simulink model "FOC IM"  (R2016a)
settings: Solver=VariableStepAuto  StartTime=0.0  StopTime=inf  FixedStep=0.000000001  RelTol=1e-4  SampleTimeConstraint=Specified
InitFcn:
  | P=2;
  | f=50;
  | we=2*pi*f;
  | rs=1.77;
  | lls=0.0139;
  | rr=1.34;
  | llr=0.0121;
  | tow=llr/rr;
  | lm=0.3687;
  | lad=1/(1/lm+1/lls+1/llr);
  | laq=lad;
  | Tl=0.1;
  | B=0.0000;
  | J=0.001;
  | Vdc=1000;
libraries: simulink x3
settings Model: Creator=moham  LastModifiedBy=moham
settings SolverCC: AutoInsertRateTranBlk=on
settings DataIOCC: ReturnWorkspaceOutputs=on
settings DebuggingCC: ArtificialAlgebraicLoopMsg=none  SFUnexpectedBacktrackingDiag=error  SFNoUnconditionalDefaultTransitionDiag=error
settings SFSimCC: SimUseLocalCustomCode=on
settings RTWCC: RTWUseLocalCustomCode=on
settings GRTTargetCC: TargetLangStandard=C99 (ISO)
settings ConfigComp: CovMetricSettings=dwe  CovSaveCumulativeToWorkspaceVar=off  CovSaveSingleToWorkspaceVar=off  CovExternalEMLEnable=on

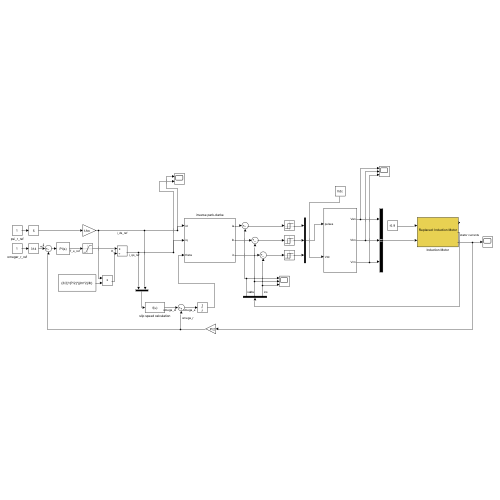
[thumbnail: Simulink's stored preview of the top-level diagram]
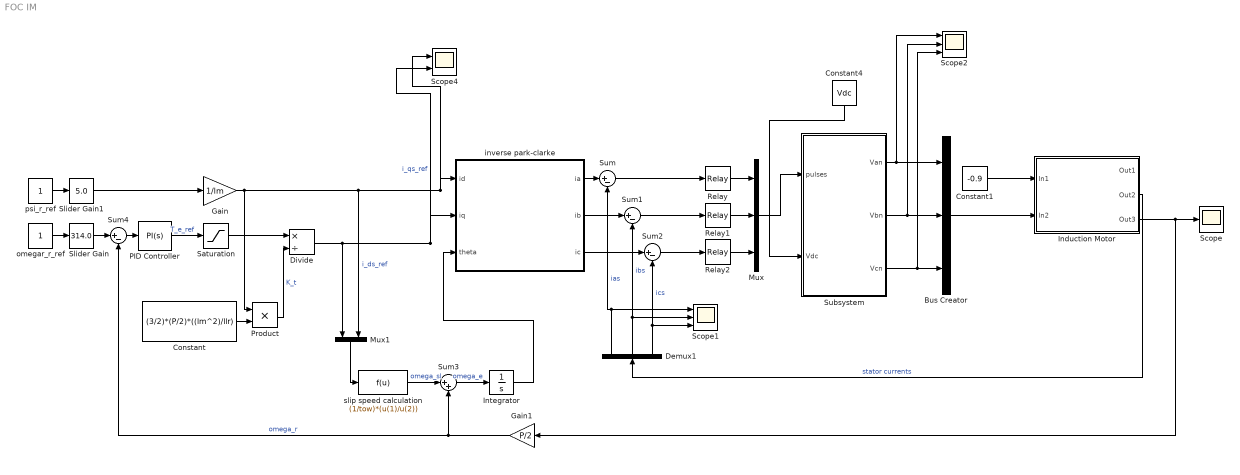
== system FOC IM ==
  Bus Creator : BusCreator  Inputs=3
  Constant : Constant  Value=(3/2)*(P/2)*((lm^2)/llr)
  Constant1 : Constant  Value=-0.9
  Constant4 : Constant  Value=Vdc
  Demux1 : Demux  Outputs=3
  Divide : Product  Inputs=*/
  Gain : Gain  Gain=1/lm
  Gain1 : Gain  Gain=P/2
  Induction Motor : Subsystem  Description=Replaced Block  mask(Replaced Block){}
      mask help: This block has been replaced with an empty subsystem because it used functionality that is unavailable in Simulink R2016a.
      mask Display: fprintf('Replaced: %s\n','Induction Motor')
  Integrator : Integrator
  Mux : Mux  Inputs=3
  Mux1 : Mux  Inputs=2
  PID Controller : simulink/Continuous/PID Controller  Controller=PI  Form=Parallel  TimeDomain=Continuous-time  SampleTime=-1  IntegratorMethod=Forward Euler  FilterMethod=Forward Euler  ControllerParametersSource=internal  P=30  I=40  D=20  N=100  UseFilter=on  InitialConditionSource=internal  InitialConditionForIntegrator=0  InitialConditionForFilter=0  DifferentiatorICPrevScaledInput=0  ExternalReset=none  TrackingMode=off  Kt=1  LimitOutput=off  UpperSaturationLimit=inf  LowerSaturationLimit=-inf  LinearizeAsGain=on  AntiWindupMode=none  Kb=1  POutMin=[]  POutMax=[]  IOutMin=[]  IOutMax=[]  DOutMin=[]  DOutMax=[]  NOutMin=[]  NOutMax=[]  SumOutMin=[]  SumOutMax=[]  SaturationOutMin=[]  SaturationOutMax=[]  PParamMin=[]  PParamMax=[]  IParamMin=[]  IParamMax=[]  DParamMin=[]  DParamMax=[]  NParamMin=[]  NParamMax=[]  KbParamMin=[]  KbParamMax=[]  KtParamMin=[]  KtParamMax=[]  KbOutMin=[]  KbOutMax=[]  KtOutMin=[]  KtOutMax=[]  IntegratorOutMin=[]  IntegratorOutMax=[]  FilterOutMin=[]  FilterOutMax=[]  SumI1OutMin=[]  SumI1OutMax=[]  SumI2OutMin=[]  SumI2OutMax=[]  SumI3OutMin=[]  SumI3OutMax=[]  SumDOutMin=[]  SumDOutMax=[]  DifferentiatorOutMin=[]  DifferentiatorOutMax=[]  IntegratorContinuousStateAttributes=''  IntegratorStateMustResolveToSignalObject=off  IntegratorRTWStateStorageClass=Auto  FilterContinuousStateAttributes=''  FilterStateMustResolveToSignalObject=off  FilterRTWStateStorageClass=Auto
  Product : Product
  Relay : Relay  OnSwitchValue=0.1  OffSwitchValue=-0.1  OffOutputValue=-1
  Relay1 : Relay  OnSwitchValue=0.1  OffSwitchValue=-0.1  OffOutputValue=-1
  Relay2 : Relay  OnSwitchValue=0.1  OffSwitchValue=-0.1  OffOutputValue=-1
  Saturation : Saturate  UpperLimit=100  LowerLimit=-100
  Scope : Scope
  Scope1 : Scope  NumInputPorts=3
  Scope2 : Scope  NumInputPorts=3
  Scope4 : Scope  NumInputPorts=2
  Slider Gain : simulink/Math Operations/Slider Gain  gain=314.0  low=-314  high=314
  Slider Gain1 : simulink/Math Operations/Slider Gain  gain=5.0  low=-5  high=5
  Subsystem : Subsystem
  Sum{,1..2,4} (4 alike) : Sum  Inputs=|+-
  Sum3 : Sum  Inputs=|++
  inverse park-clarke : Subsystem
  omegar_r_ref : Constant
  psi_r_ref : Constant
  slip speed calculation : Fcn  Expr=(1/tow)*(u(1)/u(2))
  wires:
  Sum/1 -> Relay/1
  Sum1/1 -> Relay1/1
  Sum2/1 -> Relay2/1
  inverse park-clarke/1(ia) -> Sum/1
  inverse park-clarke/3(ic) -> Sum2/1
  Constant4/1 -> Subsystem/2(Vdc)
  Mux/1 -> Subsystem/1(pulses)
  Induction Motor/2(Out2) -> Demux1/1  "stator currents"
  Demux1/1 -> Sum/2, Scope1/1  "ias"
  Demux1/2 -> Scope1/2, Sum1/2  "ibs"
  Demux1/3 -> Scope1/3, Sum2/2  "ics"
  Bus Creator/1 -> Induction Motor/2(In2)
  Induction Motor/3(Out3) -> Scope/1, Gain1/1
  Relay/1 -> Mux/1
  Relay2/1 -> Mux/3
  Relay1/1 -> Mux/2
  Constant1/1 -> Induction Motor/1(In1)
  inverse park-clarke/2(ib) -> Sum1/1
  omegar_r_ref/1 -> Slider Gain/1
  PID Controller/1 -> Saturation/1  "T_e_ref"
  Divide/1 -> Scope4/2, inverse park-clarke/2(iq), Mux1/1  "i_qs_ref"
  Constant/1 -> Product/2
  Product/1 -> Divide/2  "K_t"
  psi_r_ref/1 -> Slider Gain1/1
  Slider Gain1/1 -> Gain/1
  Gain/1 -> Scope4/1, inverse park-clarke/1(id), Mux1/2, Product/1  "i_ds_ref"
  Mux1/1 -> slip speed calculation/1
  slip speed calculation/1 -> Sum3/1  "omega_sl"
  Gain1/1 -> Sum4/2, Sum3/2  "omega_r"
  Sum3/1 -> Integrator/1  "omega_e"
  Integrator/1 -> inverse park-clarke/3(theta)
  Sum4/1 -> PID Controller/1
  Slider Gain/1 -> Sum4/1
  Saturation/1 -> Divide/1
  Subsystem/3(Vcn) -> Scope2/3, Bus Creator/3
  Subsystem/2(Vbn) -> Scope2/2, Bus Creator/2
  Subsystem/1(Van) -> Bus Creator/1, Scope2/1

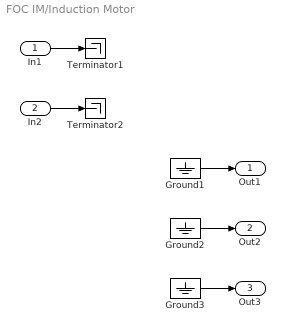
== system FOC IM/Induction Motor ==
  In1 : Inport
  In2 : Inport  Port=2
  Ground1 : Ground
  Ground2 : Ground
  Ground3 : Ground
  Terminator1 : Terminator
  Terminator2 : Terminator
  Out1 : Outport
  Out2 : Outport  Port=2
  Out3 : Outport  Port=3
  wires:
  Ground3/1 -> Out3/1
  Ground2/1 -> Out2/1
  Ground1/1 -> Out1/1
  In2/1 -> Terminator2/1
  In1/1 -> Terminator1/1

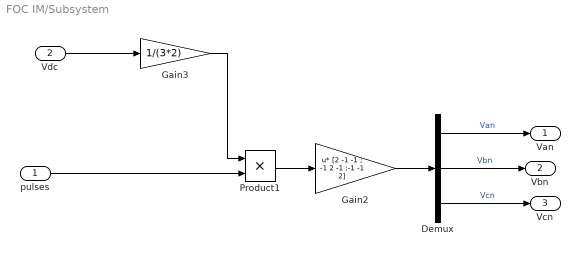
== system FOC IM/Subsystem ==
  pulses : Inport
  Vdc : Inport  Port=2
  Demux : Demux  Outputs=3
  Gain2 : Gain  Gain=[2 -1 -1 ; -1 2 -1 ;-1 -1 2]  Multiplication=Matrix(u*K)
  Gain3 : Gain  Gain=1/(3*2)
  Product1 : Product
  Van : Outport
  Vbn : Outport  Port=2
  Vcn : Outport  Port=3
  wires:
  Demux/3 -> Vcn/1  "Vcn"
  Product1/1 -> Gain2/1
  Demux/2 -> Vbn/1  "Vbn"
  Vdc/1 -> Gain3/1
  Demux/1 -> Van/1  "Van"
  Gain2/1 -> Demux/1
  Gain3/1 -> Product1/1
  pulses/1 -> Product1/2

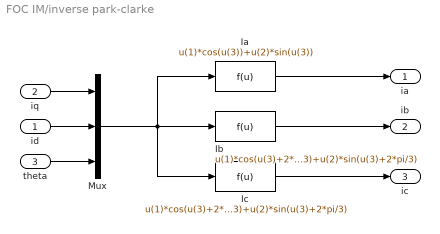
== system FOC IM/inverse park-clarke ==
  id : Inport
  iq : Inport  Port=2
  theta : Inport  Port=3
  Ia : Fcn  Expr=u(1)*cos(u(3))+u(2)*sin(u(3))
  Ib : Fcn  Expr=u(1)*cos(u(3)+2*pi/3)+u(2)*sin(u(3)+2*pi/3)
  Ic : Fcn  Expr=u(1)*cos(u(3)+2*pi/3)+u(2)*sin(u(3)+2*pi/3)
  Mux : Mux  Inputs=3
  ia : Outport
  ib : Outport  Port=2
  ic : Outport  Port=3
  wires:
  iq/1 -> Mux/1
  id/1 -> Mux/2
  theta/1 -> Mux/3
  Mux/1 -> Ic/1, Ib/1, Ia/1
  Ib/1 -> ib/1
  Ic/1 -> ic/1
  Ia/1 -> ia/1
